simulink model "Lcontainer_simNN"  (R2018b)
settings: Solver=FixedStepAuto  StartTime=0.0  StopTime=600  FixedStep=0.1  RelTol=1e-3
libraries: neural x88, simulink x1
(part 4 of 4)

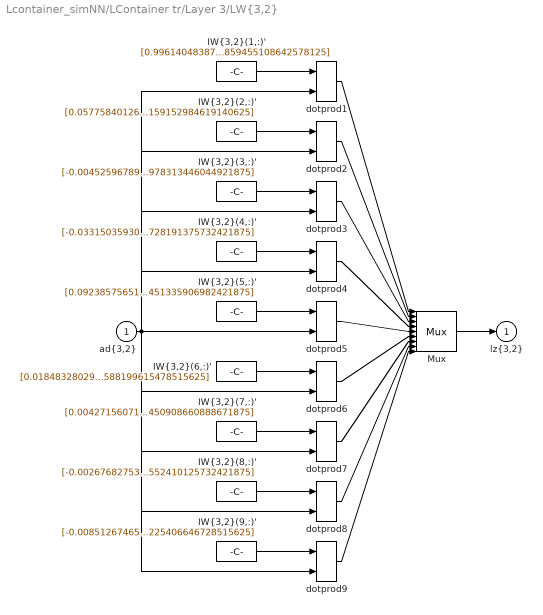
== system Lcontainer_simNN/LContainer tr/Layer 3/LW{3,2} ==
  "ad{3,2}" : Inport  PortDimensions=10
      mask Display: e = 0.06;c1 = [120 230 180]/255;c2 = ([120 230 180]+0)/(256+128);c3 = ([120 230 180]+128)/(256+128);patch([0 1 1 0],[0 0 1 1],c1);patch([0 1 1 1-e 1-e 0+e],[0 0 1 1-e 0+e 0+e],c2);patch([0 0 1 1-e 0+e 0+e],[0 1 1 1-e 1-e 0+e],c3);plot([0 1 1 0 0],[0 0 1 1 0]);
  "IW{3,2}(1,:)'" : Constant  Value=[0.99614048387105980086886347635299898684024810791015625;0.363023929990787974642074686926207505166530609130859375;-0.343901845093615710080570124773657880723476409912109375;8.7638733559965797636541148286914992837637328193522989749908447265625e-09;-5.95096160895335287531059294263702241778446477837860584259033203125e-07;0.049496405859119629866427203523926436901092529296875;-3.405311198213077777458400604258803578971992465085349977016448974609375e-09;-0.055540613694110403664172537219201331026852130889892578125;-0.20492212532710019079473795500234700739383697509765625;0.00545488178912620531868515882933934335596859455108642578125]
      mask Display: e = 0.06;c1 = [120 150 230]/255;c2 = ([120 150 230]+0)/383;c3 = ([120 150 230]+128)/383;patch([0 1 1 0],[0 0 1 1],c1);patch([0 1 1 1-e 1-e 0+e],[0 0 1 1-e 0+e 0+e],c2);patch([0 0 1 1-e 0+e 0+e],[0 1 1 1-e 1-e 0+e],c3);plot([0 1 1 0 0],[0 0 1 1 0]);disp('weights');
  "IW{3,2}(2,:)'" : Constant  Value=[0.05775840126833130250272319017312838695943355560302734375;-0.1648902809768569566184481800519279204308986663818359375;0.1527983564990939846506279309323872439563274383544921875;-5.1933398383714326322722543345135337578000189751037396490573883056640625e-09;-7.946810771813367713155111526912577346593025140464305877685546875e-06;-0.021708289150470329309516870353036210872232913970947265625;7.9954941587253634657087085317594965516718730214051902294158935546875e-08;0.0112540506464024782362631782461903640069067478179931640625;-0.079379064371409790989986277054413221776485443115234375;0.00730758983239854220670395079650916159152984619140625]
      mask Display: e = 0.06;c1 = [120 150 230]/255;c2 = ([120 150 230]+0)/383;c3 = ([120 150 230]+128)/383;patch([0 1 1 0],[0 0 1 1],c1);patch([0 1 1 1-e 1-e 0+e],[0 0 1 1-e 0+e 0+e],c2);patch([0 0 1 1-e 0+e 0+e],[0 1 1 1-e 1-e 0+e],c3);plot([0 1 1 0 0],[0 0 1 1 0]);disp('weights');
  "IW{3,2}(3,:)'" : Constant  Value=[-0.004525967896238508418604862271195088396780192852020263671875;0.006086922157890794875256812446195908705703914165496826171875;-0.006742602880192583199303602015106662292964756488800048828125;3.307571000769162053536362848847086903791847589673125185072422027587890625e-09;-2.2394736019626764115370530505710888746762066148221492767333984375e-07;0.0034200520500563334584664954007848791661672294139862060546875;-4.54143924891327704984866133145079113153652627943301922641694545745849609375e-10;-0.0064508256683157051691868133502794080413877964019775390625;0.003551391022311640478792416075748406001366674900054931640625;0.000305128602094733333664755559055947742308489978313446044921875]
      mask Display: e = 0.06;c1 = [120 150 230]/255;c2 = ([120 150 230]+0)/383;c3 = ([120 150 230]+128)/383;patch([0 1 1 0],[0 0 1 1],c1);patch([0 1 1 1-e 1-e 0+e],[0 0 1 1-e 0+e 0+e],c2);patch([0 0 1 1-e 0+e 0+e],[0 1 1 1-e 1-e 0+e],c3);plot([0 1 1 0 0],[0 0 1 1 0]);disp('weights');
  "IW{3,2}(4,:)'" : Constant  Value=[-0.033150359306823327931734723961199051700532436370849609375;0.09249785902920214242239893565056263469159603118896484375;0.1463702163257593891199093150135013274848461151123046875;-1.907724975502676457223079741344455573237581802459317259490489959716796875e-09;5.826579156795576994371833878805233553066500462591648101806640625e-06;0.725240835873029343616735786781646311283111572265625;-1.08532628109996863551195534045197554906536652197246439754962921142578125e-09;0.261274929176159298460646596140577457845211029052734375;0.369553694206814331568722309384611435234546661376953125;-0.0022431313500172636414553561934326353366486728191375732421875]
      mask Display: e = 0.06;c1 = [120 150 230]/255;c2 = ([120 150 230]+0)/383;c3 = ([120 150 230]+128)/383;patch([0 1 1 0],[0 0 1 1],c1);patch([0 1 1 1-e 1-e 0+e],[0 0 1 1-e 0+e 0+e],c2);patch([0 0 1 1-e 0+e 0+e],[0 1 1 1-e 1-e 0+e],c3);plot([0 1 1 0 0],[0 0 1 1 0]);disp('weights');
  "IW{3,2}(5,:)'" : Constant  Value=[0.09238575651210371997290593526486190967261791229248046875;0.07739798895626613661757886575287557207047939300537109375;0.4042565314884913885151718204724602401256561279296875;-6.266945374037412329289244668282903016898188752747955732047557830810546875e-10;1.000908310542831325810658911479311683478954364545643329620361328125e-06;-0.534892565735380021152423068997450172901153564453125;-3.595376058188030543334393429144406340025597046405891887843608856201171875e-09;-0.3365819156170555270790600843611173331737518310546875;0.6952711449274582289348245467408560216426849365234375;-0.0038676198652556506400734814832276242668740451335906982421875]
      mask Display: e = 0.06;c1 = [120 150 230]/255;c2 = ([120 150 230]+0)/383;c3 = ([120 150 230]+128)/383;patch([0 1 1 0],[0 0 1 1],c1);patch([0 1 1 1-e 1-e 0+e],[0 0 1 1-e 0+e 0+e],c2);patch([0 0 1 1-e 0+e 0+e],[0 1 1 1-e 1-e 0+e],c3);plot([0 1 1 0 0],[0 0 1 1 0]);disp('weights');
  "IW{3,2}(6,:)'" : Constant  Value=[0.0184832802925577188712935594594455324113368988037109375;-0.04580196366817317066288950400121393613517284393310546875;0.1178294592619949232581433307132101617753505706787109375;1.764333644896948443724692413814812697037126554278074763715267181396484375e-09;-2.00410961583632544189860491545829290771507658064365386962890625e-06;-0.014067846907664195710285781615311861969530582427978515625;3.298607848868820775983809272767499631839882567874155938625335693359375e-08;0.0102671860563745102890020888253275188617408275604248046875;-0.07527594217836053314130140279303304851055145263671875;0.002932736429353565744959642103140140534378588199615478515625]
      mask Display: e = 0.06;c1 = [120 150 230]/255;c2 = ([120 150 230]+0)/383;c3 = ([120 150 230]+128)/383;patch([0 1 1 0],[0 0 1 1],c1);patch([0 1 1 1-e 1-e 0+e],[0 0 1 1-e 0+e 0+e],c2);patch([0 0 1 1-e 0+e 0+e],[0 1 1 1-e 1-e 0+e],c3);plot([0 1 1 0 0],[0 0 1 1 0]);disp('weights');
  "IW{3,2}(7,:)'" : Constant  Value=[0.00427156071819568584901904984008069732226431369781494140625;-0.006531615910899300596337280211400866392068564891815185546875;0.00763393026123828331852561035475446260534226894378662109375;-8.89510779285081613296045266632561254738220668514259159564971923828125e-09;1.08192110116862441374620954002809536387275102242711000144481658935546875e-08;-0.004538696635365896230041027337165360222570598125457763671875;2.7568512757153752008826858173849705391234010676271282136440277099609375e-09;0.00894464854732150184413175253439476364292204380035400390625;-0.0035706280209141477537115871854211945901624858379364013671875;0.00023966576076072071237177407709850740502588450908660888671875]
      mask Display: e = 0.06;c1 = [120 150 230]/255;c2 = ([120 150 230]+0)/383;c3 = ([120 150 230]+128)/383;patch([0 1 1 0],[0 0 1 1],c1);patch([0 1 1 1-e 1-e 0+e],[0 0 1 1-e 0+e 0+e],c2);patch([0 0 1 1-e 0+e 0+e],[0 1 1 1-e 1-e 0+e],c3);plot([0 1 1 0 0],[0 0 1 1 0]);disp('weights');
  "IW{3,2}(8,:)'" : Constant  Value=[-0.002676827537542223085786918801431966130621731281280517578125;-0.047720536613422008531681939302870887331664562225341796875;-0.12419996730743891599768602418407681398093700408935546875;3.15051403747607675359430511033615764093784861188396462239325046539306640625e-10;-8.582228441747982301723482977118262482463251217268407344818115234375e-07;0.126421740899503698418726571617298759520053863525390625;1.5212950516068302102714083243011067292371762960101477801799774169921875e-08;-0.25146510340426520002665711217559874057769775390625;0.04010570207478890425445428036255179904401302337646484375;-0.0044196855292804419768071255703034694306552410125732421875]
      mask Display: e = 0.06;c1 = [120 150 230]/255;c2 = ([120 150 230]+0)/383;c3 = ([120 150 230]+128)/383;patch([0 1 1 0],[0 0 1 1],c1);patch([0 1 1 1-e 1-e 0+e],[0 0 1 1-e 0+e 0+e],c2);patch([0 0 1 1-e 0+e 0+e],[0 1 1 1-e 1-e 0+e],c3);plot([0 1 1 0 0],[0 0 1 1 0]);disp('weights');
  "IW{3,2}(9,:)'" : Constant  Value=[-0.00851267465686893730347772901723146787844598293304443359375;-0.11274536224723406829806293671936145983636379241943359375;-0.60884740537593995401977053916198201477527618408203125;-9.721720666860163526546174877032181760316831287127570249140262603759765625e-10;-7.79057722621528673709843937356112064662738703191280364990234375e-06;0.265046013500072119573047757512540556490421295166015625;6.48593176587294998580962394896243239372779498808085918426513671875e-08;-0.439981673505668469115192920071422122418880462646484375;0.330436044470342527024087075915304012596607208251953125;-0.0036704604759406644388930462952203015447594225406646728515625]
      mask Display: e = 0.06;c1 = [120 150 230]/255;c2 = ([120 150 230]+0)/383;c3 = ([120 150 230]+128)/383;patch([0 1 1 0],[0 0 1 1],c1);patch([0 1 1 1-e 1-e 0+e],[0 0 1 1-e 0+e 0+e],c2);patch([0 0 1 1-e 0+e 0+e],[0 1 1 1-e 1-e 0+e],c3);plot([0 1 1 0 0],[0 0 1 1 0]);disp('weights');
  Mux : Mux  Inputs=9
      mask Display: e = 0.06;c1 = [120 150 230]/255;c2 = ([120 150 230]+0)/383;c3 = ([120 150 230]+128)/383;patch([0 1 1 0],[0 0 1 1],c1);patch([0 1 1 1-e 1-e 0+e],[0 0 1 1-e 0+e 0+e],c2);patch([0 0 1 1-e 0+e 0+e],[0 1 1 1-e 1-e 0+e],c3);plot([0 1 1 0 0],[0 0 1 1 0]);disp('Mux');
  dotprod{1..9} (9 alike) : neural/Weight Functions/dotprod
  "lz{3,2}" : Outport
      mask Display: e = 0.06;c1 = [120 230 180]/255;c2 = ([120 230 180]+0)/(256+128);c3 = ([120 230 180]+128)/(256+128);patch([0 1 1 0],[0 0 1 1],c1);patch([0 1 1 1-e 1-e 0+e],[0 0 1 1-e 0+e 0+e],c2);patch([0 0 1 1-e 0+e 0+e],[0 1 1 1-e 1-e 0+e],c3);plot([0 1 1 0 0],[0 0 1 1 0]);
  wires:
  Mux/1 -> "lz{3,2}"/1
  dotprod9/1 -> Mux/9
  "IW{3,2}(9,:)'"/1 -> dotprod9/1
  dotprod8/1 -> Mux/8
  "IW{3,2}(8,:)'"/1 -> dotprod8/1
  dotprod7/1 -> Mux/7
  "IW{3,2}(7,:)'"/1 -> dotprod7/1
  dotprod6/1 -> Mux/6
  "IW{3,2}(6,:)'"/1 -> dotprod6/1
  dotprod5/1 -> Mux/5
  "IW{3,2}(5,:)'"/1 -> dotprod5/1
  dotprod4/1 -> Mux/4
  "IW{3,2}(4,:)'"/1 -> dotprod4/1
  dotprod3/1 -> Mux/3
  "IW{3,2}(3,:)'"/1 -> dotprod3/1
  dotprod2/1 -> Mux/2
  "IW{3,2}(2,:)'"/1 -> dotprod2/1
  dotprod1/1 -> Mux/1
  "ad{3,2}"/1 -> dotprod9/2, dotprod8/2, dotprod7/2, dotprod6/2, dotprod5/2, dotprod4/2, dotprod3/2, dotprod2/2, dotprod1/2
  "IW{3,2}(1,:)'"/1 -> dotprod1/1
